simulink model "pid_controller"  (Simulink 6.3)
settings: Solver=ode45  StartTime=0.0  StopTime=10  MaxStep=0.1  MinStep=0.001  RelTol=0.001  AbsTol=0.01
libraries: fuzblock x1
settings Model: LastModifiedBy=Administrator
settings SolverCC: InitialStep=0.001
settings OptimizationCC: BooleanDataType=off
settings DebuggingCC: SolverPrmCheckMsg=none
settings HardwareCC: TargetUnknown=on

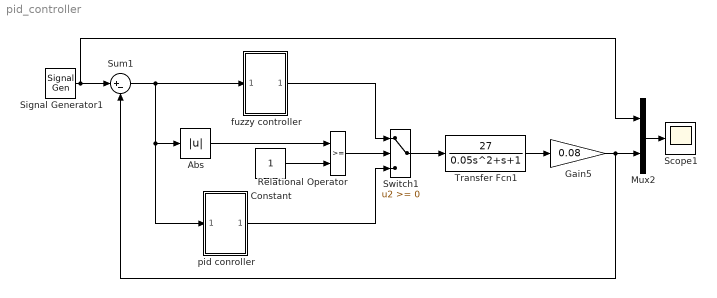
== system pid_controller ==
  Abs : Abs  SaturateOnIntegerOverflow=on
  Constant : Constant
  Gain5 : Gain  Gain=0.08  SaturateOnIntegerOverflow=on
  Mux2 : Mux  Inputs=2
  Relational Operator : RelationalOperator  InputSameDT=on
  Scope1 : Scope
      settings: TimeRange=1.5  YMin=0.7475  YMax=0.805  SaveName=ScopeData2
  Signal Generator1 : SignalGenerator  Units=rad/sec
  Sum1 : Sum  Inputs=|+-  SaturateOnIntegerOverflow=on  InputSameDT=on
  Switch1 : Switch
  Transfer Fcn1 : TransferFcn  Numerator=[27]  Denominator=[0.05 1 1]
  fuzzy controller : Subsystem
  pid conroller : Subsystem
  wires:
  Constant/1 -> Relational Operator/2
  Abs/1 -> Relational Operator/1
  Gain5/1 -> Mux2/2, Sum1/2
  Mux2/1 -> Scope1/1
  Relational Operator/1 -> Switch1/2
  Sum1/1 -> Abs/1, pid conroller/1(In1), fuzzy controller/1(In1)
  Signal Generator1/1 -> Sum1/1, Mux2/1
  pid conroller/1(Out1) -> Switch1/3
  Transfer Fcn1/1 -> Gain5/1
  fuzzy controller/1(Out1) -> Switch1/1
  Switch1/1 -> Transfer Fcn1/1

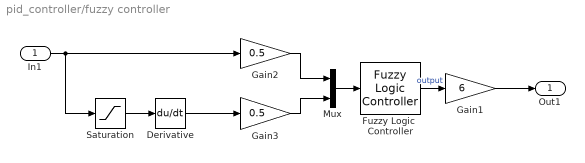
== system pid_controller/fuzzy controller ==
  In1 : Inport
  Derivative : Derivative
  Fuzzy Logic  Controller : fuzblock/Fuzzy Logic  Controller  fis=fuzzy
  Gain1 : Gain  Gain=6  SaturateOnIntegerOverflow=on
  Gain2 : Gain  Gain=0.5  SaturateOnIntegerOverflow=on
  Gain3 : Gain  Gain=0.5  SaturateOnIntegerOverflow=on
  Mux : Mux  Inputs=2
  Saturation : Saturate  UpperLimit=10  LowerLimit=-10
  Out1 : Outport
  wires:
  Derivative/1 -> Gain3/1
  Saturation/1 -> Derivative/1
  In1/1 -> Saturation/1, Gain2/1
  Mux/1 -> Fuzzy Logic  Controller/1
  Fuzzy Logic  Controller/1 -> Gain1/1  "output"
  Gain3/1 -> Mux/2
  Gain2/1 -> Mux/1
  Gain1/1 -> Out1/1

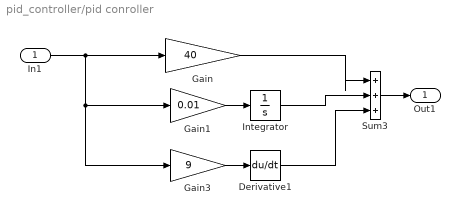
== system pid_controller/pid conroller ==
  In1 : Inport
  Derivative1 : Derivative
  Gain : Gain  Gain=40  SaturateOnIntegerOverflow=on
  Gain1 : Gain  Gain=0.01  SaturateOnIntegerOverflow=on
  Gain3 : Gain  Gain=9  SaturateOnIntegerOverflow=on
  Integrator : Integrator
  Sum3 : Sum  Inputs=|+++  SaturateOnIntegerOverflow=on  InputSameDT=on
  Out1 : Outport
  wires:
  Gain1/1 -> Integrator/1
  Gain3/1 -> Derivative1/1
  Gain/1 -> Sum3/1
  Derivative1/1 -> Sum3/3
  In1/1 -> Gain/1, Gain1/1, Gain3/1
  Integrator/1 -> Sum3/2
  Sum3/1 -> Out1/1
